simulink model "pidsimutt"  (R2020b)
settings: Solver=ode23  StartTime=0.0  StopTime=1000  MaxStep=1  MinStep=0.001  RelTol=1e-2  EnableMultiTasking=on
settings Model: Creator=pptt  LastModifiedBy=ThinkPad
settings SolverCC: InitialStep=0.01
settings DataIOCC: LimitDataPoints=on  SaveFormat=Array  SignalLoggingSaveFormat=ModelDataLogs  ReturnWorkspaceOutputs=off  SignalLoggingName=sigsOut  Refine=3
settings OptimizationCC: OptimizeBlockIOStorage=off  BufferReuse=off  GlobalBufferReuse=off  ExpressionFolding=off  LocalBlockOutputs=off  InitFltsAndDblsToZero=on  LifeSpan=inf
settings DebuggingCC: SaveWithParameterizedLinksMsg=none  UnderspecifiedInitializationDetection=Classic  MergeDetectMultiDrivingBlocksExec=none  SignalResolutionControl=TryResolveAllWithWarning  MultiTaskDSMMsg=warning  MultiTaskCondExecSysMsg=none  SFUnexpectedBacktrackingDiag=warning  SFNoUnconditionalDefaultTransitionDiag=warning  SFExecutionAtInitializationDiag=none  ArithmeticOperatorsInVariantConditions=warning
settings HardwareCC: ProdBitPerPointer=32  ProdBitPerSizeT=32  ProdBitPerPtrDiffT=32  ProdLargestAtomicFloat=None  ProdIntDivRoundTo=Undefined  ProdEndianess=Unspecified  ProdWordSize=32  ProdHWDeviceType=32-bit Generic  TargetUnknown=on
settings ModelReferenceCC: PropagateSignalLabelsOutOfModel=off
settings SFSimCC: SimUseLocalCustomCode=off  CustomCodeUndefinedFunction=UseInterfaceOnly
settings RTWCC: RTWUseLocalCustomCode=off
settings CodeAppCC: StateflowObjectComments=on
settings GRTTargetCC: TargetFcnLib=ansi_tfl_tmw.mat  TargetLangStandard=C89/C90 (ANSI)  CombineOutputUpdateFcns=off  GRTInterface=on
settings ConfigComp: CovMetricSettings=dw  CovSaveCumulativeToWorkspaceVar=on  CovSaveSingleToWorkspaceVar=on  CovExternalEMLEnable=off

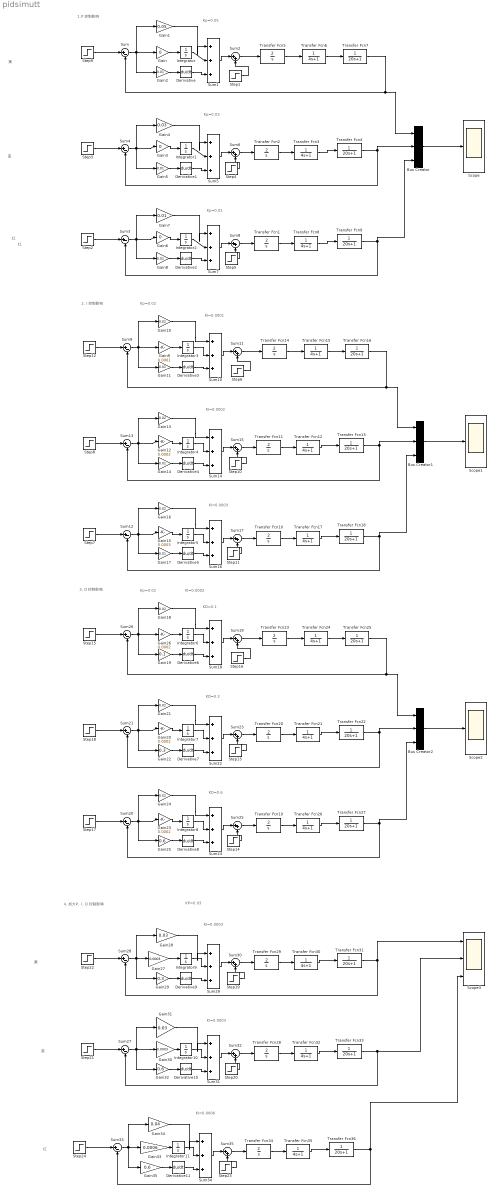
== system pidsimutt ==
  note: 蓝
  note: Kp=0.05
  note: 1,P 控制影响
  note: Kp=0.03
  note: Kp=0.01
  note: 2, I 控制影响
  note: KI=0.0003
  note: KI=0.0002
  note: KI=0.0001
  note: Kp=0.02
  note: KD=0.3
  note: KI=0.0002
  note: Kp=0.02
  note: KD=0.6
  note: 3, D 控制影响
  note: KD=0.1
  note: KI=0.0003
  note: KI=0.0003
  note: 4, 加大P、I, D 控制影响
  note: KP=0.03
  note: 黄
  note: 红
  note: KI=0.0006
  note: 红
  note: 红
  note: 蓝
  note: 黄
  Bus Creator : BusCreator  Inputs=3
  Bus Creator1 : BusCreator  Inputs=3
  Bus Creator2 : BusCreator  Inputs=3
  Derivative{,1..11} (12 alike) : Derivative
  Gain : Gain  Gain=0  SaturateOnIntegerOverflow=on  OutDataTypeStr=Inherit: Same as input  ParamDataTypeStr=Inherit: Same as input
  Gain1 : Gain  Gain=0.05  SaturateOnIntegerOverflow=on  OutDataTypeStr=Inherit: Same as input  ParamDataTypeStr=Inherit: Same as input
  Gain{10,13,16,18,21,24} (6 alike) : Gain  Gain=0.02  SaturateOnIntegerOverflow=on  OutDataTypeStr=Inherit: Same as input  ParamDataTypeStr=Inherit: Same as input
  Gain{2,5,7..8,11,14,17} (7 alike) : Gain  Gain=0.01  SaturateOnIntegerOverflow=on  OutDataTypeStr=Inherit: Same as input  ParamDataTypeStr=Inherit: Same as input
  Gain{12,20,23,26} (4 alike) : Gain  Gain=0.0002  SaturateOnIntegerOverflow=on  OutDataTypeStr=Inherit: Same as input  ParamDataTypeStr=Inherit: Same as input
  Gain15 : Gain  Gain=0.0003  SaturateOnIntegerOverflow=on  OutDataTypeStr=Inherit: Same as input  ParamDataTypeStr=Inherit: Same as input
  Gain19 : Gain  Gain=0.1  SaturateOnIntegerOverflow=on  OutDataTypeStr=Inherit: Same as input  ParamDataTypeStr=Inherit: Same as input
  Gain22 : Gain  Gain=0.3  SaturateOnIntegerOverflow=on  OutDataTypeStr=Inherit: Same as input  ParamDataTypeStr=Inherit: Same as input
  Gain25 : Gain  Gain=0.6  SaturateOnIntegerOverflow=on  OutDataTypeStr=Inherit: Same as input  ParamDataTypeStr=Inherit: Same as input
  Gain27 : Gain  Gain=0.0003  SaturateOnIntegerOverflow=on  OutDataTypeStr=Inherit: Same as input  ParamDataTypeStr=Inherit: Same as input
  Gain28 : Gain  Gain=0.03  SaturateOnIntegerOverflow=on  OutDataTypeStr=Inherit: Same as input  ParamDataTypeStr=Inherit: Same as input
  Gain29 : Gain  Gain=0.3  SaturateOnIntegerOverflow=on  OutDataTypeStr=Inherit: Same as input  ParamDataTypeStr=Inherit: Same as input
  Gain3 : Gain  Gain=0  SaturateOnIntegerOverflow=on  OutDataTypeStr=Inherit: Same as input  ParamDataTypeStr=Inherit: Same as input
  Gain30 : Gain  Gain=0.0003  SaturateOnIntegerOverflow=on  OutDataTypeStr=Inherit: Same as input  ParamDataTypeStr=Inherit: Same as input
  Gain31 : Gain  Gain=0.03  SaturateOnIntegerOverflow=on  OutDataTypeStr=Inherit: Same as input  ParamDataTypeStr=Inherit: Same as input
  Gain32 : Gain  Gain=0.6  SaturateOnIntegerOverflow=on  OutDataTypeStr=Inherit: Same as input  ParamDataTypeStr=Inherit: Same as input
  Gain33 : Gain  Gain=0.0006  SaturateOnIntegerOverflow=on  OutDataTypeStr=Inherit: Same as input  ParamDataTypeStr=Inherit: Same as input
  Gain34 : Gain  Gain=0.04  SaturateOnIntegerOverflow=on  OutDataTypeStr=Inherit: Same as input  ParamDataTypeStr=Inherit: Same as input
  Gain35 : Gain  Gain=0.6  SaturateOnIntegerOverflow=on  OutDataTypeStr=Inherit: Same as input  ParamDataTypeStr=Inherit: Same as input
  Gain4 : Gain  Gain=0.03  SaturateOnIntegerOverflow=on  OutDataTypeStr=Inherit: Same as input  ParamDataTypeStr=Inherit: Same as input
  Gain6 : Gain  Gain=0  SaturateOnIntegerOverflow=on  OutDataTypeStr=Inherit: Same as input  ParamDataTypeStr=Inherit: Same as input
  Gain9 : Gain  Gain=0.0001  SaturateOnIntegerOverflow=on  OutDataTypeStr=Inherit: Same as input  ParamDataTypeStr=Inherit: Same as input
  Integrator{,1..11} (12 alike) : Integrator
  Scope : Scope
  Scope1 : Scope
  Scope2 : Scope
  Scope3 : Scope  NumInputPorts=3
  Step{1,4..6,10..11,13..14,16,19..20,23} (12 alike) : Step  Time=500  After=0.02  SampleTime=1
  Step{2..3,7..9,12,15,17..18,21..22,24} (12 alike) : Step  Time=0  SampleTime=1
  Sum{,3..4,9,12..13,20..21,26..28,33} (12 alike) : Sum  Inputs=|+-  SaturateOnIntegerOverflow=on
  Sum{1,5,7,10,14,16,18,22,24,29,31,34} (12 alike) : Sum  Inputs=|+++  SaturateOnIntegerOverflow=on
  Sum{2,6,8,11,15,17,19,23,25,30,32,35} (12 alike) : Sum  Inputs=|++  SaturateOnIntegerOverflow=on
  Transfer Fcn{1..2,5,10..11,14,19..20,23,28..29,34} (12 alike) : TransferFcn  Numerator=[2]  Denominator=[1 0]
  Transfer Fcn{3,6,8,12,15,17,21,24,26,30,32,35} (12 alike) : TransferFcn  Denominator=[4 1]
  Transfer Fcn{4,7,9,13,16,18,22,25,27,31,33,36} (12 alike) : TransferFcn  Denominator=[20 1]
  wires:
  Sum/1 -> Gain/1, Gain2/1, Gain1/1
  Gain1/1 -> Sum1/1
  Gain/1 -> Integrator/1
  Integrator/1 -> Sum1/2
  Gain2/1 -> Derivative/1
  Derivative/1 -> Sum1/3
  Sum1/1 -> Sum2/1
  Step3/1 -> Sum4/1
  Sum4/1 -> Gain3/1, Gain5/1, Gain4/1
  Gain4/1 -> Sum5/1
  Gain3/1 -> Integrator1/1
  Integrator1/1 -> Sum5/2
  Gain5/1 -> Derivative1/1
  Derivative1/1 -> Sum5/3
  Sum5/1 -> Sum6/1
  Sum6/1 -> Transfer Fcn2/1
  Step4/1 -> Sum6/2
  Step9/1 -> Sum/1
  Step1/1 -> Sum2/2
  Transfer Fcn4/1 -> Bus Creator/2, Sum4/2
  Transfer Fcn3/1 -> Transfer Fcn4/1
  Transfer Fcn5/1 -> Transfer Fcn6/1
  Transfer Fcn6/1 -> Transfer Fcn7/1
  Sum2/1 -> Transfer Fcn5/1
  Transfer Fcn7/1 -> Sum/2, Bus Creator/1
  Transfer Fcn2/1 -> Transfer Fcn3/1
  Bus Creator/1 -> Scope/1
  Transfer Fcn1/1 -> Transfer Fcn8/1
  Transfer Fcn8/1 -> Transfer Fcn9/1
  Sum7/1 -> Sum8/1
  Integrator2/1 -> Sum7/2
  Sum3/1 -> Gain6/1, Gain8/1, Gain7/1
  Derivative2/1 -> Sum7/3
  Gain7/1 -> Sum7/1
  Step2/1 -> Sum3/1
  Gain8/1 -> Derivative2/1
  Gain6/1 -> Integrator2/1
  Sum8/1 -> Transfer Fcn1/1
  Step5/1 -> Sum8/2
  Transfer Fcn9/1 -> Bus Creator/3, Sum3/2
  Transfer Fcn11/1 -> Transfer Fcn12/1
  Sum11/1 -> Transfer Fcn14/1
  Transfer Fcn10/1 -> Transfer Fcn17/1
  Transfer Fcn18/1 -> Bus Creator1/3, Sum12/2
  Step11/1 -> Sum17/2
  Sum17/1 -> Transfer Fcn10/1
  Gain17/1 -> Derivative5/1
  Gain16/1 -> Sum16/1
  Sum16/1 -> Sum17/1
  Transfer Fcn15/1 -> Transfer Fcn16/1
  Transfer Fcn14/1 -> Transfer Fcn15/1
  Bus Creator1/1 -> Scope1/1
  Transfer Fcn16/1 -> Sum9/2, Bus Creator1/1
  Gain9/1 -> Integrator3/1
  Derivative5/1 -> Sum16/3
  Integrator4/1 -> Sum14/2
  Gain10/1 -> Sum10/1
  Derivative3/1 -> Sum10/3
  Step12/1 -> Sum9/1
  Sum13/1 -> Gain12/1, Gain14/1, Gain13/1
  Transfer Fcn17/1 -> Transfer Fcn18/1
  Step6/1 -> Sum11/2
  Derivative4/1 -> Sum14/3
  Sum12/1 -> Gain15/1, Gain17/1, Gain16/1
  Sum15/1 -> Transfer Fcn11/1
  Sum10/1 -> Sum11/1
  Sum14/1 -> Sum15/1
  Sum9/1 -> Gain9/1, Gain11/1, Gain10/1
  Gain14/1 -> Derivative4/1
  Gain13/1 -> Sum14/1
  Step8/1 -> Sum13/1
  Gain15/1 -> Integrator5/1
  Gain11/1 -> Derivative3/1
  Transfer Fcn12/1 -> Transfer Fcn13/1
  Integrator5/1 -> Sum16/2
  Gain12/1 -> Integrator4/1
  Step10/1 -> Sum15/2
  Integrator3/1 -> Sum10/2
  Transfer Fcn13/1 -> Bus Creator1/2, Sum13/2
  Step7/1 -> Sum12/1
  Step17/1 -> Sum20/1
  Gain21/1 -> Sum22/1
  Gain19/1 -> Derivative6/1
  Step13/1 -> Sum23/2
  Integrator6/1 -> Sum18/2
  Gain23/1 -> Integrator8/1
  Sum20/1 -> Gain23/1, Gain25/1, Gain24/1
  Sum22/1 -> Sum23/1
  Gain22/1 -> Derivative7/1
  Sum23/1 -> Transfer Fcn20/1
  Sum26/1 -> Gain26/1, Gain19/1, Gain18/1
  Step16/1 -> Sum19/2
  Sum18/1 -> Sum19/1
  Transfer Fcn22/1 -> Bus Creator2/2, Sum21/2
  Sum21/1 -> Gain20/1, Gain22/1, Gain21/1
  Step18/1 -> Sum21/1
  Derivative6/1 -> Sum18/3
  Step15/1 -> Sum26/1
  Transfer Fcn24/1 -> Transfer Fcn25/1
  Integrator8/1 -> Sum24/2
  Bus Creator2/1 -> Scope2/1
  Derivative8/1 -> Sum24/3
  Transfer Fcn21/1 -> Transfer Fcn22/1
  Gain18/1 -> Sum18/1
  Integrator7/1 -> Sum22/2
  Gain26/1 -> Integrator6/1
  Transfer Fcn25/1 -> Sum26/2, Bus Creator2/1
  Transfer Fcn26/1 -> Transfer Fcn27/1
  Transfer Fcn27/1 -> Bus Creator2/3, Sum20/2
  Gain24/1 -> Sum24/1
  Sum25/1 -> Transfer Fcn19/1
  Step14/1 -> Sum25/2
  Gain25/1 -> Derivative8/1
  Sum24/1 -> Sum25/1
  Transfer Fcn19/1 -> Transfer Fcn26/1
  Transfer Fcn23/1 -> Transfer Fcn24/1
  Gain20/1 -> Integrator7/1
  Sum19/1 -> Transfer Fcn23/1
  Derivative7/1 -> Sum22/3
  Transfer Fcn20/1 -> Transfer Fcn21/1
  Sum28/1 -> Gain27/1, Gain29/1, Gain28/1
  Transfer Fcn30/1 -> Transfer Fcn31/1
  Transfer Fcn31/1 -> Scope3/1, Sum28/2
  Step22/1 -> Sum28/1
  Sum30/1 -> Transfer Fcn29/1
  Sum29/1 -> Sum30/1
  Sum27/1 -> Gain30/1, Gain32/1, Gain31/1
  Gain30/1 -> Integrator10/1
  Gain31/1 -> Sum31/1
  Gain28/1 -> Sum29/1
  Step19/1 -> Sum30/2
  Integrator10/1 -> Sum31/2
  Transfer Fcn33/1 -> Scope3/2, Sum27/2
  Derivative9/1 -> Sum29/3
  Transfer Fcn28/1 -> Transfer Fcn32/1
  Gain27/1 -> Integrator9/1
  Gain32/1 -> Derivative10/1
  Integrator9/1 -> Sum29/2
  Sum32/1 -> Transfer Fcn28/1
  Derivative10/1 -> Sum31/3
  Step20/1 -> Sum32/2
  Gain29/1 -> Derivative9/1
  Transfer Fcn32/1 -> Transfer Fcn33/1
  Sum31/1 -> Sum32/1
  Transfer Fcn29/1 -> Transfer Fcn30/1
  Step21/1 -> Sum27/1
  Integrator11/1 -> Sum34/2
  Derivative11/1 -> Sum34/3
  Gain33/1 -> Integrator11/1
  Sum34/1 -> Sum35/1
  Sum35/1 -> Transfer Fcn34/1
  Gain34/1 -> Sum34/1
  Transfer Fcn36/1 -> Scope3/3, Sum33/2
  Sum33/1 -> Gain34/1, Gain33/1, Gain35/1
  Transfer Fcn34/1 -> Transfer Fcn35/1
  Step23/1 -> Sum35/2
  Step24/1 -> Sum33/1
  Transfer Fcn35/1 -> Transfer Fcn36/1
  Gain35/1 -> Derivative11/1
